simulink library "lib_decmp_Calib_tbm_brkBts_x8"  (R2020a)
settings: Solver=VariableStepAuto  StartTime=0.0  StopTime=10.0  RelTol=1e-3
settings Model: Creator=Administrator  LastModifiedBy=Administrator

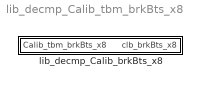
== system lib_decmp_Calib_tbm_brkBts_x8 ==
  lib_decmp_Calib_brkBts_x8 : Subsystem

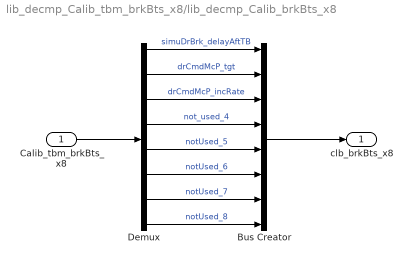
== system lib_decmp_Calib_tbm_brkBts_x8/lib_decmp_Calib_brkBts_x8 ==
  Calib_tbm_brkBts_x8 : Inport  OutDataTypeStr=single  PortDimensions=8
  Bus Creator : BusCreator  Inputs=8
  Demux : Demux  Outputs=8
  clb_brkBts_x8 : Outport  PortDimensions=8
  wires:
  Calib_tbm_brkBts_x8/1 -> Demux/1
  Demux/1 -> Bus Creator/1  "simuDrBrk_delayAftTB"
  Demux/2 -> Bus Creator/2  "drCmdMcP_tgt"
  Demux/3 -> Bus Creator/3  "drCmdMcP_incRate"
  Demux/4 -> Bus Creator/4  "not_used_4"
  Bus Creator/1 -> clb_brkBts_x8/1
  Demux/5 -> Bus Creator/5  "notUsed_5"
  Demux/6 -> Bus Creator/6  "notUsed_6"
  Demux/7 -> Bus Creator/7  "notUsed_7"
  Demux/8 -> Bus Creator/8  "notUsed_8"
